simulink model "Model_I6_CoM_Earth_Axes"  (Simulink 6.6)
settings: Solver=ode45  StartTime=tmin  StopTime=tmax  MaxStep=dt  RelTol=1e-3
values from neighbouring files (symbols this model uses):
  dt = 0.01    [Pgm_G11_Superposition.m]    (also in Pgm_G12_Num_Integration.m; Pgm_G13_Frequency_Domain.m = 0.0625; Pgm_H2_Response_Gusts_Control.m = 0.001; Pgm_H3_Ase_Gusts_Pid.m = 0.001)
settings Model: Creator=Jan Wright  LastModifiedBy=Jan Wright
settings DataIOCC: SignalLoggingName=sigsOut
settings DebuggingCC: SignalResolutionControl=TryResolveAllWithWarning  SolverPrmCheckMsg=none  MultiTaskDSMMsg=warning  MultiTaskCondExecSysMsg=none  StrictBusMsg=None
settings HardwareCC: TargetUnknown=on
settings RTWCC: IncludeERTFirstTime=on
settings GRTTargetCC: ModelReferenceCompliant=off  MatFileLogging=off

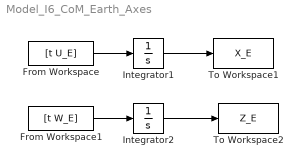
== system Model_I6_CoM_Earth_Axes ==
  From Workspace : FromWorkspace  VariableName=[t U_E]  SampleTime=dt
  From Workspace1 : FromWorkspace  VariableName=[t W_E]  SampleTime=dt
  Integrator1 : Integrator
  Integrator2 : Integrator
  To Workspace1 : ToWorkspace  VariableName=X_E  SampleTime=dt  SaveFormat=Array
  To Workspace2 : ToWorkspace  VariableName=Z_E  SampleTime=dt  SaveFormat=Array
  wires:
  From Workspace/1 -> Integrator1/1
  Integrator1/1 -> To Workspace1/1
  From Workspace1/1 -> Integrator2/1
  Integrator2/1 -> To Workspace2/1
